simulink model "Lab1_Water_Tank_Temperature_Heating_Coil"  (R2017b)
settings: Solver=VariableStepAuto  StartTime=0.0  StopTime=60  RelTol=1e-3
settings Model: Creator=hxa134  LastModifiedBy=Joseph

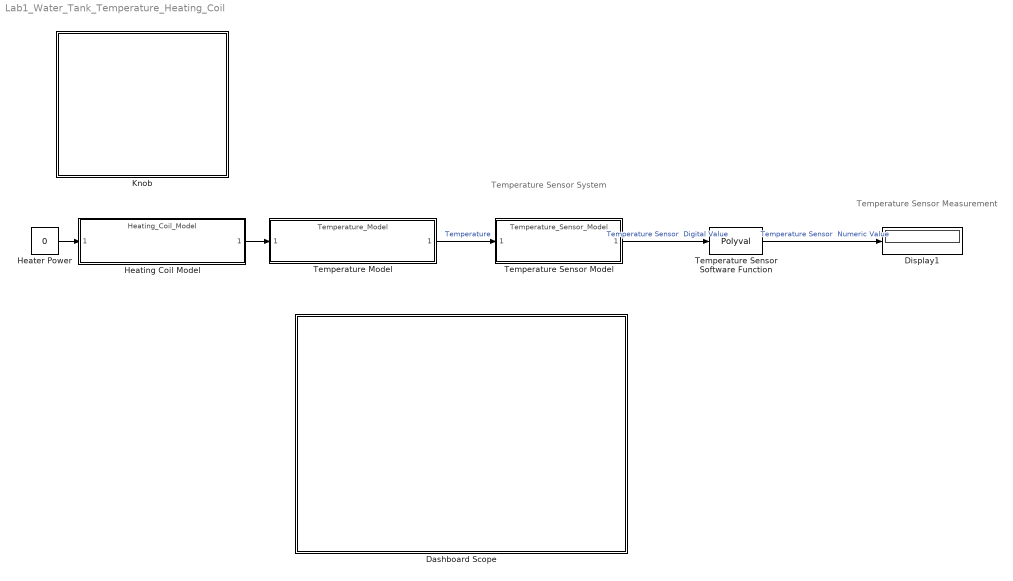
== system Lab1_Water_Tank_Temperature_Heating_Coil ==
  note: Temperature Sensor System
  note: Temperature Sensor Measurement
  Dashboard Scope : Subsystem  DialogController=hmiCreateDDGDialog  IsWebBlock=on  mask(MWDashboardBlock){webBlockId=2a1a89e9-3606-4793-9b6e-01017e02ca12, webBlockType=sdiscope, ShowInitialText=on, HMISrcModelName=Lab1_Water_Tank_Temperature_Heating_Coil}
      mask prompts: webBlockId "WebBlock Id"; webBlockType "WebBlock Type"; HMISrcModelName "Source Model"
      mask help: SimulinkHMI:dialogs:HMIScopeDialogDesc
      mask Help: helpview([docroot '/mapfiles/simulink.map'], 'hmi_scope')
      mask Display:
      | if strcmp(get_param(bdroot(gcb),'BlockDiagramType'), 'library')
      |     image([(matlabroot) '/toolbox/simulink/hmi/icons/DashboardScope.png']);
      | end
  Display1 : Display
  Heater Power : Constant  Value=0
  Heating Coil Model : ModelReference  ModelNameDialog=Heating_Coil_Model  ModelReferenceVersion=1.24  CopyOfModelProtected=on
  Knob : Subsystem  DialogController=hmiCreateDDGDialog  IsWebBlock=on  mask(MWDashboardBlock){webBlockId=f1d15619-c2b9-4264-80fc-b36746c0ed4a, webBlockType=continuousknob, ShowInLibBrowser=on, ShowInitialText=on, HMISrcModelName=Lab1_Water_Tank_Temperature_Heating_Coil}
      mask prompts: webBlockId "WebBlock Id"; webBlockType "WebBlock Type"; HMISrcModelName "Source Model"
      mask help: SimulinkHMI:dialogs:ContinuousKnobDialogDesc
      mask Help: helpview([docroot '/mapfiles/simulink.map'], 'hmi_knob')
      mask Display:
      | if strcmp(get_param(bdroot(gcb),'BlockDiagramType'), 'library')
      |     image([(matlabroot) '/toolbox/simulink/hmi/icons/ContinuousKnob.png']);
      | end
  Temperature Model : ModelReference  ModelNameDialog=Temperature_Model.slxp  ModelReferenceVersion=1.24  CopyOfModelProtected=on
  Temperature Sensor Software Function : Polyval  Coefs="[2.0008   -0.0067]"
  Temperature Sensor Model : ModelReference  ModelNameDialog=Temperature_Sensor_Model.slxp  ModelReferenceVersion=1.24  CopyOfModelProtected=on
  wires:
  Heater Power/1 -> Heating Coil Model/1
  Temperature Sensor Model/1 -> Temperature Sensor Software Function/1  "Temperature Sensor  Digital Value"
  Temperature Sensor Software Function/1 -> Display1/1  "Temperature Sensor  Numeric Value"
  Temperature Model/1 -> Temperature Sensor Model/1  "Temperature"
  Heating Coil Model/1 -> Temperature Model/1

== system Lab1_Water_Tank_Temperature_Heating_Coil/Dashboard Scope ==

== system Lab1_Water_Tank_Temperature_Heating_Coil/Knob ==
